simulink model "r"  (Simulink 8.7)
settings: Solver=VariableStepAuto  StartTime=0.0  StopTime=10.0  RelTol=1e-3
settings Model: Creator=yyy  LastModifiedBy=yyy
settings DataIOCC: LimitDataPoints=off  SaveFormat=Dataset
settings DebuggingCC: UnderspecifiedInitializationDetection=Simplified  MergeDetectMultiDrivingBlocksExec=error
settings HardwareCC: ProdBitPerPointer=64  ProdLargestAtomicFloat=Float  ProdIntDivRoundTo=Zero  ProdEndianess=LittleEndian  ProdWordSize=64  ProdHWDeviceType=Intel->x86-64 (Windows64)
settings ModelReferenceCC: PropagateSignalLabelsOutOfModel=on
settings ConfigComp: CovModelRefEnable=off

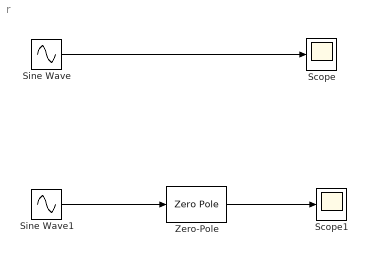
== system r ==
  Scope : Scope
  Scope1 : Scope
  Sine Wave : Sin  Amplitude=2  Bias=0.5  Frequency=0.4*pi  SampleTime=0
  Sine Wave1 : Sin  Amplitude=2  Bias=0.5  Frequency=0.4*pi  SampleTime=0
  Zero-Pole : ZeroPole  Zeros=[0]  Poles=[-2]
  wires:
  Sine Wave/1 -> Scope/1
  Sine Wave1/1 -> Zero-Pole/1
  Zero-Pole/1 -> Scope1/1
